simulink model "FIR_Filter"  (R2019b)
settings: Solver=VariableStepAuto  StartTime=0.0  StopTime=10.0  RelTol=1e-3
settings Model: Creator=ip  LastModifiedBy=ip

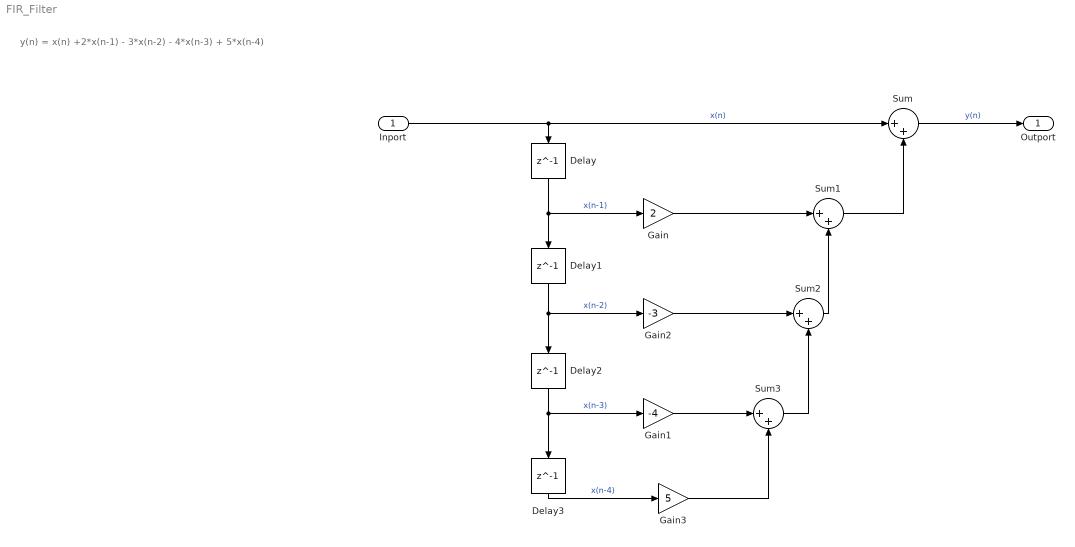
== system FIR_Filter ==
  note: y(n) = x(n) +2*x(n-1) - 3*x(n-2) - 4*x(n-3) + 5*x(n-4)
  Inport : Inport
  Delay{,1..3} (4 alike) : Delay  DelayLength=1
  Gain : Gain  Gain=2
  Gain1 : Gain  Gain=-4
  Gain2 : Gain  Gain=-3
  Gain3 : Gain  Gain=5
  Sum{,1..3} (4 alike) : Sum  Inputs=|++
  Outport : Outport
  wires:
  Inport/1 -> Sum/1, Delay/1  "x(n)"
  Sum/1 -> Outport/1  "y(n)"
  Delay/1 -> Delay1/1, Gain/1  "x(n-1)"
  Delay1/1 -> Delay2/1, Gain2/1  "x(n-2)"
  Delay2/1 -> Delay3/1, Gain1/1  "x(n-3)"
  Gain/1 -> Sum1/1
  Gain2/1 -> Sum2/1
  Gain1/1 -> Sum3/1
  Delay3/1 -> Gain3/1  "x(n-4)"
  Gain3/1 -> Sum3/2
  Sum3/1 -> Sum2/2
  Sum2/1 -> Sum1/2
  Sum1/1 -> Sum/2
